simulink model "prob01"  (Simulink 7.4)
settings: Solver=ode45  StartTime=0.0  StopTime=40  RelTol=1e-3
libraries: cstblocks x4, dspsrcs4 x1
settings Model: Creator=AshfaqAhmad  LastModifiedBy=AshfaqAhmad

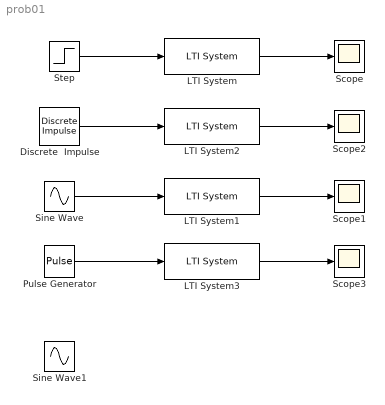
== system prob01 ==
  Discrete  Impulse : dspsrcs4/Discrete  Impulse  Delay=0  SampleTime=1  FrameSample=1  dataType=double  isSigned=on  wordLen=16  udDataType=sfix(16)  fracBitsMode=Best precision  numFracBits=15
  LTI System{,1..3} (4 alike) : cstblocks/LTI System  SystemSampleTime=-1  sys=tf(100,[1 4 20])  IC=[]
  Pulse Generator : DiscretePulseGenerator  PulseType=Time based  Amplitude=2  Period=10  PulseWidth=5  PhaseDelay=0  SampleTime=1
  Scope{,1..3} (4 alike) : Scope
      Scope2 settings: SaveName=ScopeData2
      Scope3 settings: SaveName=ScopeData3
  Sine Wave : Sin  Amplitude=1  Bias=0  Frequency=1  Phase=0  Samples=10  SampleTime=0  Offset=0
  Sine Wave1 : Sin  Amplitude=1  Bias=0  Frequency=1  Phase=0  Samples=10  SampleTime=0  Offset=0
  Step : Step  SampleTime=0
  wires:
  Step/1 -> LTI System/1
  LTI System/1 -> Scope/1
  Sine Wave/1 -> LTI System1/1
  LTI System1/1 -> Scope1/1
  Discrete  Impulse/1 -> LTI System2/1
  LTI System2/1 -> Scope2/1
  Pulse Generator/1 -> LTI System3/1
  LTI System3/1 -> Scope3/1
